simulink model "thrust_vector_rocket"  (R2024b)
settings: Solver=VariableStepAuto  StartTime=0.0  StopTime=15.0  RelTol=1e-3
libraries: simulink x1, simulink_extras x1
settings Model: Creator=wolfl  LastModifiedBy=wolfl

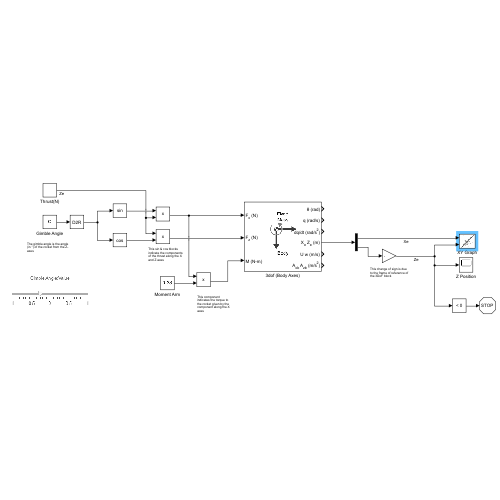
[thumbnail: Simulink's stored preview of the top-level diagram]
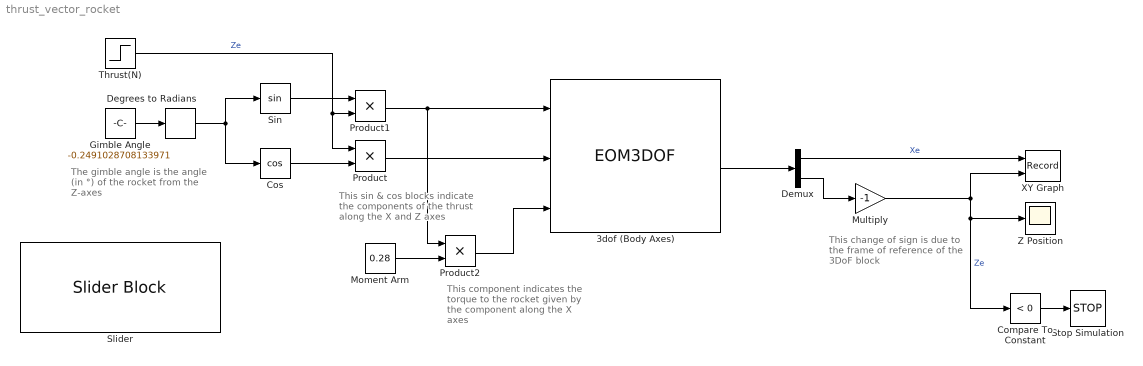
== system thrust_vector_rocket ==
  note: This component indicates the torque to the rocket given by the component along the X axes
  note: This sin & cos blocks indicate the components of the thrust along the X and Z axes
  note: The gimble angle is the angle (in °) of the rocket from the Z-axes
  note: This change of sign is due to the frame of reference of the 3DoF block
  3dof (Body Axes) : EOM3DOF  v_ini=0  mass=0.543  Iyy=0.048
  Compare To Constant : simulink/Logic and Bit Operations/Compare To Constant  relop=<  const=0  OutDataTypeStr=boolean
  Cos : Trigonometry  Operator=cos
  Degrees to Radians : simulink_extras/Transformations/Degrees to Radians
  Demux : Demux  Outputs=2
  Gimble Angle : Constant  Value=-0.2491028708133971
  Moment Arm : Constant  Value=0.28
  Multiply : Gain  Gain=-1
  Product : Product
  Product1 : Product
  Product2 : Product
  Sin : Trigonometry
  Slider : SliderBlock  ScaleMin=-1  ScaleMax=1  TickInterval=0.5
  Stop Simulation : Stop
  Thrust(N) : Step  Time=2  Before=-15  After=0  SampleTime=0
  XY Graph : Record  FileSettingsInternal="{\"entries\":[{\"content\":{\"excelSettings\":{\"content\":{},\"type\":\"Streamout.ExcelSettings\"}},\"type\":\"Streamout.FileSettingStorage\",\"uuid\":\"\"}],\"packageUris\":[\"http:\\/\\/schema.mathworks.com\\/mf0\\/streamout_blocks\\/R2020a\"],\"version\":\"1.0\"}"  Layout=[1 1]  SignalsInternal="{\"entries\":[{\"content\":{\"signals\":[{\"content\":{\"blockPath\":[],\"dimensions\":[1],\"domain\":\"\",\"lineColor\":\"#a2142f\",\"plots\":[ 1 ],\"port\":1,\"sid\":[\"\"],\"signalID\":1,\"signalName\":\"Xe\"},\"type\":\"RecordBlkView.Signal\",\"uuid\":\"\"},{\"content\":{\"blockPath\":[],\"dimensions\":[1],\"domain\":\"\",\"lineColor\":\"#139fff\",\"plots\":[ 1 ],\"port\":2,\"sid\":[\"\"],\"signalID\":2,\"signalName\":\"Ze\"},\"type\":\"RecordBlkView.Signal\",\"uuid\":\"\"}]},\"type\":\"RecordBlkView.InputSignals\",\"uuid\":\"\"}],\"packageUris\":[\"http:\\/\\/schema.mathworks.com\\/mf0\\/streamout_blocks\\/R2020a\"],\"version\":\"1.0\"}"  VisualizationBindings="{\"xyplotplugin\":{\"info\":[{\"series\":[{\"bindingParametersList\":[{\"parameter\":\"X-Axis\",\"signalID\":1,\"signalName\":\"Xe\"},{\"parameter\":\"Y-Axis\",\"signalID\":2,\"signalName\":\"Ze\"}],\"seriesID\":0}],\"subplotID\":1}]}}"  CompatibilityTag=XY
  Z Position : Scope
  wires:
  3dof (Body Axes)/4 -> Demux/1
  Demux/2 -> Multiply/1
  Demux/1 -> XY Graph/1  "Xe"
  Multiply/1 -> XY Graph/2, Compare To Constant/1, Z Position/1  "Ze"
  Compare To Constant/1 -> Stop Simulation/1
  Thrust(N)/1 -> Product/1, Product1/2  "Ze"
  Gimble Angle/1 -> Degrees to Radians/1
  Degrees to Radians/1 -> Cos/1, Sin/1
  Sin/1 -> Product1/1
  Cos/1 -> Product/2
  Product/1 -> 3dof (Body Axes)/2
  Product1/1 -> Product2/1, 3dof (Body Axes)/1
  Product2/1 -> 3dof (Body Axes)/3
  Moment Arm/1 -> Product2/2
